simulink library "dspxfrm3"  (Simulink 6.0)
settings: Solver=ode45  SolverMode=SingleTasking  StartTime=0.0  StopTime=10.0  RelTol=1e-3
undefined symbols (not defined in the file or in its folder): D, dspblkDDClose, magnitude, Rows
libraries: dspmtrx3 x7, dspsigops x6, dspxfrm3 x6, dspsigattribs x5, dspbuff3 x2, dsparch4 x1, dspsrcs4 x1, simulink x1, dspspect3 x1
settings Model: RequirementInfo=9  CovMetricSettings=d  Creator=szlotkin  LastModifiedBy=mlongfri  ExtModeAutoUpdateStatusClock=off  ProdHWDeviceType=Specified
settings DataIOCC: SignalLoggingName=logsOut
settings OptimizationCC: BooleanDataType=off
settings DebuggingCC: CheckExecutionContextPreStartOutputMsg=on  CheckExecutionContextRuntimeOutputMsg=on  SolverPrmCheckMsg=none
settings HardwareCC: ProdHWDeviceType=Specified  TargetUnknown=on
settings ModelReferenceCC: UpdateModelReferenceTargets=IfOutOfDate
settings SFSimCC: SFSimApplyToAllLibs=on  SFSimBuildMode=Incremental

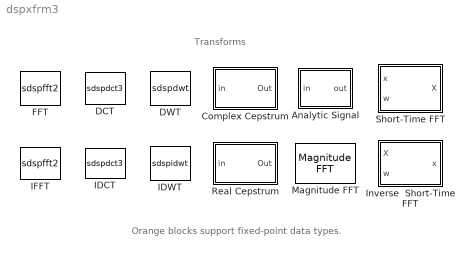
== system dspxfrm3 ==
  note: Transforms
  note: Orange blocks support fixed-point data types.
  Analytic Signal : Subsystem  PropExecContextAcrossSSBoundary=on  mask(Analytic Signal){N=100}
      mask prompts: N "Filter order (must be even):"
      mask help: Complex analytic signal of input.
      mask init:
      | x = [0,NaN,100,NaN,[58 58],NaN,[24 92],NaN,[58 24 24 58],NaN,[58 64 68 72 76 80 84 88],NaN, [42 42],NaN,[8 76],NaN,[72 68 64 60 56 52 48 42 36 32 28 24 20 16 12],NaN,[32 43 45 43 35]];
      | y = [0,NaN,100,NaN,[43 8],NaN,[16 16],NaN,[18 18 17 17],NaN,[16 24 36 24 28 28 32 16],NaN, [92 56],NaN,[64 64],NaN,[64 80 76 76 72 84 72 64 72 84 72 76 76 80 64],NaN,[51 33 41 33 35] ];
      | b=dspblkanalytic2('design',N);
      mask Help: web(dspbhelp);
      mask Display: plot(x,y)
  Complex Cepstrum : Subsystem  PropExecContextAcrossSSBoundary=on  mask(Complex Cepstrum){inheritFFT=on, N=64}
      mask prompts: inheritFFT "Inherit FFT length from input port dimensions"; N "FFT length:"
      mask help: Complex cepstrum of input signal. Input is modified to remove possible phase discontinuity at +/- pi radians.
      mask init:
      | dspblkcceps('init');
      mask Help: web(dspbhelp);
      mask CallbackString: dspblkcceps|
      mask Display: disp('Complex\n Cepstrum')
  DCT : S-Function  FunctionName=sdspdct3  Parameters=0, CompMethod  mask(DCT){CompMethod=Table lookup}
      mask prompts: CompMethod "Sine and cosine computation:"
      mask help:
      | Outputs the discrete cosine transform (DCT) of a real or complex input by computing a fast cosine transform (FCT) using a radix-2 FFT.
      |
      | Computes the DCT along the vector dimension for sample-based vector inputs, which must have a power-of-2 length. Computes the DCT along each column for all other inputs, where the columns must be a power-of-2 length.
      mask Help: web(dspbhelp);
      mask StyleString: popup(Table lookup|Trigonometric fcn)
      mask Display: disp(' DCT')
  DWT : S-Function  FunctionName=sdspdwt  Parameters=phl, phh, NumLevels, tree, Output  mask(DWT){Wname=User-defined, OrdRec_ordDec=[1 / 1], Order=2, LPF=[0.0352   -0.0854   -0.1350   0.4599   0.8069   0.3327], HPF=[-0.3327    0.8069   -0.4599   -0.1350    0.0854    0.0352], NumLevels=2, tree=Asymmetric, Output=Single port}
      mask prompts: Wname "Filter:"; OrdRec_ordDec "Filter order [synthesis / analysis]:"; Order "Wavelet order:"; LPF "Lowpass FIR filter coefficients:"; HPF "Highpass FIR filter coefficients:"; NumLevels "Number of levels:"; tree "Tree structure:"
      mask help:
      | Computes the discrete wavelet transform (DWT). Uses a filter bank with specified highpass and lowpass FIR filters to decompose the input into subbands that have smaller bandwidths and slower sample rates. The filters can be user-defined or wavelet-based (use of wavelets requires the Wavelet Toolbox).  Usually, the highpass and lowpass filters should be half-band filters designed to complement each other.
      |
      | When 'Output' is set to 'Multiple ports' the block outputs each subband from a different port as a frame-based vector or matrix (the topmost port outputs the subband with the highest frequency band). When 'Output' is set to 'Single port' the block outputs one sample-based vector or matrix of concatenated subbands.
      |
      | Inputs must be frame-based with a frame size a multiple of 2^n, where n is the value entered in the 'Number of levels.'  To create a filter bank that accepts sample-based inputs and inputs of other sizes, use Two-Channel Analysis Subband Filter blocks in the Multirate Filters library.
      |
      | This block is the same as the Dyadic Analysis Filter Bank block in the Multirate Filters library.
      mask init:
      | [x,y, str] = dspblkdwt('icon');
      | [phl, phh] = dspblkdwt('init', LPF, HPF, tree);
      mask Help: web(dspbhelp);
      mask StyleString: popup(User-defined|Haar|Daubechies|Symlets|Coiflets|Biorthogonal|Reverse Biorthogonal|Discrete Meyer),popup([1 / 1]|[1 / 3]|[1 / 5]|[2 / 2]|[2 / 4]|[2 / 6]|[2 / 8]|[3 / 1]|[3 / 3]|[3 / 5]|[3 / 7]|[3 / 9]|[4 / 4]|[5 / 5]|[6 / 8]),edit,edit,edit,edit,popup(Asymmetric|Symmetric),popup(Single port|Multiple ports)
      mask CallbackString: dspblkdwt|||||||
      mask Display:
      | disp(' DWT')
      | 
      | text(0.07,0.16,str)
  FFT : S-Function  DialogController=dspDDGCreate  DialogControllerArgs=DataTag2  FunctionName=sdspfft2  Parameters=0,CompMethod,TableOpt,BitRevOrder,0,SkipNorm,dtInfo.firstCoeffMode,dtInfo.firstCoeffWordLength,dtInfo.firstCoeffFracLength,dtInfo.prodOutputMode,dtInfo.prodOutputWordLength,dtInfo.prodOutputFracLength,dtInfo.accumMode,dtInfo.accumWordLength,dtInfo.accumFracLength,dtInfo.outputMode,dtInfo.outputWordLength,dtInfo.outputFracLength,dtInfo.roundingMode,dtInfo.overflowMode  mask(FFT){CompMethod=Table lookup, TableOpt=Speed, BitRevOrder=off, additionalParams=off, SkipNorm=on, allowOverrides=on, firstCoeffMode=Same word length as input, firstCoeffWordLength=16, firstCoeffFracLength=15, outputMode=Inherit via internal rule, outputWordLength=16, outputFracLength=15, accumMode=Inherit via internal rule, accumWordLength=32, accumFracLength=30, prodOutputMode=Inherit via internal rule, prodOutputWordLength=32, prodOutputFracLength=30, roundingMode=Floor, overflowMode=off, LockScale=off}
      mask prompts: CompMethod "Twiddle factor computation:"; TableOpt "Optimize table for:"; BitRevOrder "Output in bit-reversed order"; additionalParams "---------- Show additional parameters ----------"; SkipNorm "Skip divide-by-two on butterfly outputs for fixed-point signals"; allowOverrides "Allow overrides from DSP Fixed-Point Attributes blocks"; firstCoeffMode "Fixed-point sine table attributes:"; firstCoeffWordLength "Sine table word length:"; firstCoeffFracLength "Sine table fraction length:"; outputMode "Fixed-point output attributes:"; outputWordLength "Output word length:"; outputFracLength "Output fraction length:"; accumMode "Fixed-point accumulator attributes:"; accumWordLength "Accumulator word length:"; accumFracLength "Accumulator fraction length:"; prodOutputMode "Fixed-point product output attributes:"; prodOutputWordLength "Product output word length:"; prodOutputFracLength "Product output fraction length:"; roundingMode "Round integer calculations toward:"; overflowMode "Saturate on integer overflow"; LockScale "Lock scaling"
      mask help:
      | Outputs the complex fast Fourier transform (FFT) of a real or complex input by computing radix-2 decimation-in-time (DIT) or decimation-in-frequency (DIF), depending on block options. Uses half-length and double-signal algorithms for real inputs where possible.
      |
      | Computes the FFT along the vector dimension for sample-based vector inputs, which must have a power-of-2 length. Computes the FFT along each column for all other inputs, where the columns must be a power-of-2 length.
      mask init:
      | dtInfo = dspGetFixptDataTypeInfo(gcbh,47);
      settings: CopyFcn=dspfixptcopycallback
      mask Help: web(dspbhelp);
      mask StyleString: popup(Trigonometric fcn|Table lookup),popup(Speed|Memory),checkbox,checkbox,checkbox,checkbox,popup(Same word length as input|Specify word length|Same as input|Same as output|User-defined|Binary point scaling|Slope and bias scaling),edit,edit,popup(Inherit via internal rule|Same as input|Binary point scaling|Slope and bias scaling|User-defined),edit,edit,popup(Inherit via internal rule|Same as product output|Same as input|Binary point scaling|Slope and bias scaling|User-defined),edit,edit,popup(Inherit via internal rule|Same as input|Binary point scaling|Slope and bias scaling|User-defined),edit,edit,popup(Floor|Nearest),checkbox,checkbox
      mask Display: disp('  FFT ');
  IDCT : S-Function  FunctionName=sdspdct3  Parameters=1, CompMethod  mask(IDCT){CompMethod=Table lookup}
      mask prompts: CompMethod "Sine and cosine computation:"
      mask help:
      | Outputs the inverse discrete cosine transform (IDCT) of a real or complex input by computing an inverse fast cosine transform (IFCT) using a radix-2 IFFT.
      |
      | Computes the IDCT along the vector dimension for sample-based vector inputs, which must have a power-of-2 length. Computes the IDCT along each column for all other inputs, where the columns must be a power-of-2 length.
      mask Help: web(dspbhelp);
      mask StyleString: popup(Table lookup|Trigonometric fcn)
      mask Display: disp('IDCT')
  IDWT : S-Function  FunctionName=sdspidwt  Parameters=phl, phh, NumLevels, tree, Input  mask(IDWT){Wname=User-defined, OrdRec_ordDec=[1 / 1], Order=2, LPF=[0.3327    0.8069    0.4599   -0.1350   -0.0854    0.0352], HPF=[0.0352    0.0854   -0.1350   -0.4599    0.8069   -0.3327], NumLevels=2, tree=Asymmetric, Input=Single port}
      mask prompts: Wname "Filter:"; OrdRec_ordDec "Filter order [synthesis, analysis]:"; Order "Wavelet order:"; LPF "Lowpass FIR filter coefficients:"; HPF "Highpass FIR filter coefficients:"; NumLevels "Number of levels:"; tree "Tree Structure:"
      mask help:
      | Computes the inverse discrete wavelet transform (IDWT). Uses a filter bank with specified highpass and lowpass FIR filters to reconstruct the original signal from its subbands, which have smaller bandwidths and slower sample rates. Filters can be user-defined or wavelet-based (use of wavelets requires the Wavelet Toolbox). Usually, the highpass and lowpass filters should be half-band filters designed to complement each other.
      |
      | When 'Input' is set to 'Multiple ports', you must input each subband through a different input port as a frame-based vector or matrix (the topmost input port should receive the subband with the highest frequency band). When 'Input' is set to 'Single port', the block input must be a sample-based vector or matrix of concatenated subbands.
      |
      | To create a filter bank with less constraints on whether the inputs are frame-based or sample-based, use Two-Channel Synthesis Subband Filter blocks in the Multirate Filters library.
      |
      | This block is the same as the Dyadic Synthesis Filter Bank block in the Multirate Filters library.
      mask init:
      | [x,y,str] = dspblkidwt('icon');
      | [phl, phh] = dspblkidwt('init', LPF, HPF, tree);
      mask Help: web(dspbhelp);
      mask StyleString: popup(User-defined|Haar|Daubechies|Symlets|Coiflets|Biorthogonal|Reverse Biorthogonal|Discrete Meyer),popup([1 / 1]|[1 / 3]|[1 / 5]|[2 / 2]|[2 / 4]|[2 / 6]|[2 / 8]|[3 / 1]|[3 / 3]|[3 / 5]|[3 / 7]|[3 / 9]|[4 / 4]|[5 / 5]|[6 / 8]),edit,edit,edit,edit,popup(Asymmetric|Symmetric),popup(Single port|Multiple ports)
      mask CallbackString: dspblkidwt|||||||
      mask Display:
      | disp(' IDWT')
      | text(0.07,0.16,str)
  IFFT : S-Function  DialogController=dspDDGCreate  DialogControllerArgs=DataTag3  ClipboardFcn=dspblkDDClose;  FunctionName=sdspfft2  Parameters=1,CompMethod,TableOpt,BitRevOrder,cs_in,SkipNorm,dtInfo.firstCoeffMode,dtInfo.firstCoeffWordLength,dtInfo.firstCoeffFracLength,dtInfo.prodOutputMode,dtInfo.prodOutputWordLength,dtInfo.prodOutputFracLength,dtInfo.accumMode,dtInfo.accumWordLength,dtInfo.accumFracLength,dtInfo.outputMode,dtInfo.outputWordLength,dtInfo.outputFracLength,dtInfo.roundingMode,dtInfo.overflowMode  mask(IFFT){CompMethod=Table lookup, TableOpt=Speed, BitRevOrder=off, cs_in=off, SkipNorm=off, mode=Complex, additionalParams=off, allowOverrides=on, firstCoeffMode=Same word length as input, firstCoeffWordLength=16, firstCoeffFracLength=15, outputMode=Inherit via internal rule, outputWordLength=16, outputFracLength=15, accumMode=Inherit via internal rule, accumWordLength=32, accumFracLength=30, prodOutputMode=Inherit via internal rule, prodOutputWordLength=32, prodOutputFracLength=30, roundingMode=Floor, overflowMode=off, LockScale=off}
      mask prompts: CompMethod "Twiddle factor computation:"; TableOpt "Optimize table for:"; BitRevOrder "Input is in bit-reversed order"; cs_in "Input is conjugate symmetric"; SkipNorm "Skip scaling"; mode "Output:"; additionalParams "---------- Show additional parameters ----------"; allowOverrides "Allow overrides from DSP FPA Fixed-Point Attributes blocks"; firstCoeffMode "Fixed-point sine table attributes:"; firstCoeffWordLength "Sine table word length:"; firstCoeffFracLength "Sine table fraction length:"; outputMode "Fixed-point output attributes:"; outputWordLength "Output word length:"; outputFracLength "Output fraction length:"; accumMode "Fixed-point accumulator attributes:"; accumWordLength "Accumulator word length:"; accumFracLength "Accumulator fraction length:"; prodOutputMode "Fixed-point product output attributes:"; prodOutputWordLength "Product output word length:"; prodOutputFracLength "Product output fraction length:"; roundingMode "Round integer calculations toward:"; overflowMode "Saturate on integer overflow"; LockScale "Lock scaling"
      mask help:
      | Outputs the inverse fast Fourier transform (IFFT) of a real or complex input by computing radix-2 decimation-in-time (DIT) or decimation-in-frequency (DIF), depending on block options. Outputs are real if you select 'Input is conjugate symmetric' option; otherwise, outputs are complex.
      |
      | Computes the IFFT along the vector dimension for sample-based vector inputs, which must have a power-of-2 length. Computes the IFFT along each column for all other inputs, where the columns must be a power-of-2 length.
      mask init:
      | dtInfo = dspGetFixptDataTypeInfo(gcbh,47);
      settings: CopyFcn=dspfixptcopycallback
      mask Help: web(dspbhelp);
      mask StyleString: popup(Trigonometric fcn|Table lookup),popup(Speed|Memory),checkbox,checkbox,checkbox,popup(Real|Complex),checkbox,checkbox,popup(Same word length as input|Specify word length|Same as input|Same as output|User-defined|Binary point scaling|Slope and bias scaling),edit,edit,popup(Inherit via internal rule|Same as input|Binary point scaling|Slope and bias scaling|User-defined),edit,edit,popup(Inherit via internal rule|Same as product output|Same as input|Binary point scaling|Slope and bias scaling|User-defined),edit,edit,popup(Inherit via internal rule|Same as input|Binary point scaling|Slope and bias scaling|User-defined),edit,edit,popup(Floor|Nearest),checkbox,checkbox
      mask Display: disp('  IFFT')
  Inverse  Short-Time FFT : Subsystem  PropExecContextAcrossSSBoundary=on  mask(Inverse Short-Time FFT){OvLap=512-16, OutFrameSize=512, InConjSymm=on, DoAssert=off, W=512, Tol=1e-4}
      mask prompts: OvLap "Overlap between consecutive STFFT frames (in samples):"; OutFrameSize "Samples per output frame:"; InConjSymm "Input is conjugate symmetric"; DoAssert "Assert if analysis window does not support perfect signal reconstruction"; W "Analysis window length:"; Tol "Reconstruction error tolerance:"
      mask help:
      | Reconstructs a signal from its Short-Time FFT (STFFT) by using the OLA method. The block takes as an input the analysis window w[n] used in the generation of the STFFT to normalize the output signal.
      |
      | Optionally, the block asserts if the analysis window does not satisfy
      | constraints that permit perfect reconstruction of the signal.
      mask init:
      | L = dspblkistfft('init',DoAssert,OvLap,W,InConjSymm);
      mask Help: web(dspbhelp)
      mask CallbackString: |||dspblkistfft('dynamic');||
      mask Display:
      | port_label('input',1,'X[nL,k]')
      | port_label('output',1,'x[n]')
      | port_label('input',2,'w[n]')
  Magnitude FFT : dspspect3/Magnitude FFT  mag_or_magsq=Magnitude squared  fftLenInherit=off  fftsize=256
  Real Cepstrum : Subsystem  PropExecContextAcrossSSBoundary=on  mask(Real Cepstrum){inheritFFT=on, N=64}
      mask prompts: inheritFFT "Inherit FFT length from input port dimensions"; N "FFT length:"
      mask help: Real cepstrum of input signal.
      mask init:
      | dspblkrceps('init');
      mask Help: web(dspbhelp);
      mask CallbackString: dspblkrceps|
      mask Display: disp('Real\nCepstrum')
  Short-Time FFT : Subsystem  PropExecContextAcrossSSBoundary=on  mask(Short-Time FFT){W=512, OvLap=512-16, M=1024}
      mask prompts: W "Analysis window length:"; OvLap "Overlap between consecutive windows (in samples):"; M "FFT length:"
      mask help:
      | Output the Short-Time FFT of the input signal x[n].
      | Uses an externally specified analysis window w[n].
      mask init:
      | L = W-OvLap;
      settings: CopyFcn=dspfixptcopycallback
      mask Help: web(dspbhelp)
      mask Display:
      | port_label('input',1,'x[n]')
      | port_label('input',2,'w[n]')
      | port_label('output',1,'X[nL,k]')

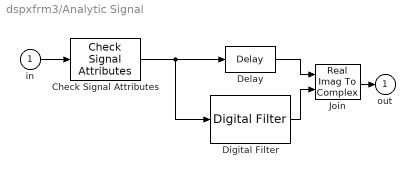
== system dspxfrm3/Analytic Signal ==
  in : Inport  LatchInput=off
  Check Signal Attributes : dspsigattribs/Check Signal Attributes  SigAttribCheckMethod=Does not match attributes exactly  Complexity=Ignore  Frame=Ignore  DimsCheckMethod=Ignore  Dimensions=1-D  DatatypeCheckMethod=Is...  DatatypeGeneral=Floating-point  DtypeFloatSpecific=Any floating-point  DtypeFixedSpecific=Any fixed-point  DtypeIntSpecific=Any integer  SampleMode=Ignore
  Delay : dspsigops/Delay  dly_unit=Samples  delay=N/2  ic_detail=off  dif_ic_for_ch=off  dif_ic_for_dly=off  ic=0  reset_popup=None
  Digital Filter : dsparch4/Digital Filter  TypePopup=FIR (all zeros)  IIRFiltStruct=Direct form II transposed  AllPoleFiltStruct=Direct form  FIRFiltStruct=Direct form transposed  CoeffSource=Specify via dialog  NumCoeffs=b  DenCoeffs=[1 0.1]  BiQuadCoeffs=[1 0.3 0.4 1 0.1 0.2]  LatticeCoeffs=[0.2 0.4]  denIgnore=on  FiltPerSampPopup=One filter per frame  IC=0  ICnum=0  ICden=0  roundingMode=Floor  overflowMode=off
  Join : RealImagToComplex
  out : Outport  InitialOutput=0
  wires:
  Digital Filter/1 -> Join/2
  Delay/1 -> Join/1
  Join/1 -> out/1
  in/1 -> Check Signal Attributes/1
  Check Signal Attributes/1 -> Delay/1, Digital Filter/1

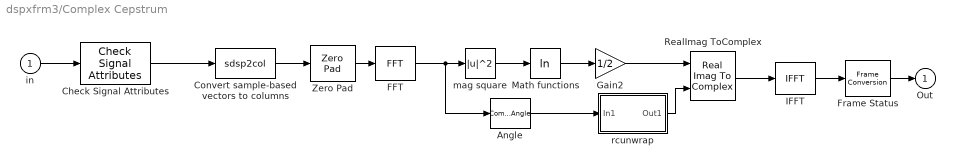
== system dspxfrm3/Complex Cepstrum ==
  in : Inport  LatchInput=off
  Angle : ComplexToMagnitudeAngle  Output=Angle
  Check Signal Attributes : dspsigattribs/Check Signal Attributes  SigAttribCheckMethod=Does not match attributes exactly  Complexity=Real  Frame=Ignore  DimsCheckMethod=Ignore  Dimensions=1-D  DatatypeCheckMethod=Is...  DatatypeGeneral=Floating-point  DtypeFloatSpecific=Any floating-point  DtypeFixedSpecific=Any fixed-point  DtypeIntSpecific=Any integer  SampleMode=Discrete
  Convert sample-based vectors to columns : S-Function  FunctionName=sdsp2col
  FFT : dspxfrm3/FFT  DialogController=dspDDGCreate  DialogControllerArgs=DataTag0  CompMethod=Table lookup  TableOpt=Speed  BitRevOrder=off  SkipNorm=on  roundingMode=Floor  overflowMode=off
  Frame Status : FrameConversion  OutFrame=Sample based
  Gain2 : Gain  Gain=1/2  SaturateOnIntegerOverflow=on
  IFFT : dspxfrm3/IFFT  DialogController=dspDDGCreate  DialogControllerArgs=DataTag1  CompMethod=Table lookup  TableOpt=Speed  BitRevOrder=off  cs_in=on  SkipNorm=off  mode=Real  roundingMode=Floor  overflowMode=off
  Math functions : Math  Operator=log  SaturateOnIntegerOverflow=on
  RealImag ToComplex : RealImagToComplex
  Zero Pad : dspsigops/Zero Pad  padSigAt=End  zpadAlong=None  padNumOutRowsSpecMethod=User-specified  numOutRows=N  padNumOutColsSpecMethod=User-specified  numOutCols=1  trunc_flag=None
  mag square : Math  Operator=magnitude^2  SaturateOnIntegerOverflow=on
  rcunwrap : Subsystem  PropExecContextAcrossSSBoundary=on
  Out : Outport  InitialOutput=0
  wires:
  Gain2/1 -> RealImag ToComplex/1
  rcunwrap/1(Out1) -> RealImag ToComplex/2
  mag square/1 -> Math functions/1
  Math functions/1 -> Gain2/1
  in/1 -> Check Signal Attributes/1
  FFT/1 -> mag square/1, Angle/1
  Angle/1 -> rcunwrap/1(In1)
  IFFT/1 -> Frame Status/1
  Convert sample-based vectors to columns/1 -> Zero Pad/1
  Zero Pad/1 -> FFT/1
  Frame Status/1 -> Out/1
  RealImag ToComplex/1 -> IFFT/1
  Check Signal Attributes/1 -> Convert sample-based vectors to columns/1

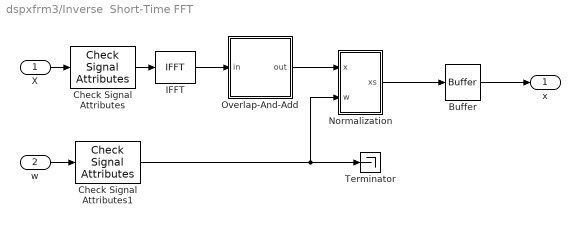
== system dspxfrm3/Inverse  Short-Time FFT ==
  X : Inport  LatchInput=off
  w : Inport  Port=2  LatchInput=off
  Buffer : dspbuff3/Buffer  N=OutFrameSize  V=0  ic=0
  Check Signal Attributes : dspsigattribs/Check Signal Attributes  SigAttribCheckMethod=Does not match attributes exactly  Complexity=Ignore  Frame=Ignore  DimsCheckMethod=Ignore  Dimensions=1-D  DatatypeCheckMethod=Is...  DatatypeGeneral=Floating-point  DtypeFloatSpecific=Any floating-point  DtypeFixedSpecific=Any fixed-point  DtypeIntSpecific=Any integer  SampleMode=Ignore
  Check Signal Attributes1 : dspsigattribs/Check Signal Attributes  SigAttribCheckMethod=Does not match attributes exactly  Complexity=Ignore  Frame=Ignore  DimsCheckMethod=Ignore  Dimensions=1-D  DatatypeCheckMethod=Is...  DatatypeGeneral=Floating-point  DtypeFloatSpecific=Any floating-point  DtypeFixedSpecific=Any fixed-point  DtypeIntSpecific=Any integer  SampleMode=Ignore
  IFFT : dspxfrm3/IFFT  DialogController=dspDDGCreate  DialogControllerArgs=DataTag4  CompMethod=Table lookup  TableOpt=Speed  BitRevOrder=off  cs_in=on  SkipNorm=off  mode=Real  roundingMode=Floor  overflowMode=off
  Normalization : Subsystem  PropExecContextAcrossSSBoundary=on
  Overlap-And-Add : Subsystem  PropExecContextAcrossSSBoundary=on  mask(Overlap-And-Add){L=L}
      mask prompts: L "Number of new points in each frame"
      mask help: Performs overlap-and-add on the input signal. Disjoint frames of the input signal are overlapped with each other for a specified number of points and summed.
      mask Display: disp('Overlap\nAnd\nAdd')
  Terminator : Terminator
  x : Outport
  wires:
  Normalization/1(xs) -> Buffer/1
  IFFT/1 -> Overlap-And-Add/1(in)
  Overlap-And-Add/1(out) -> Normalization/1(x)
  X/1 -> Check Signal Attributes/1
  w/1 -> Check Signal Attributes1/1
  Buffer/1 -> x/1
  Check Signal Attributes/1 -> IFFT/1
  Check Signal Attributes1/1 -> Normalization/2(w), Terminator/1

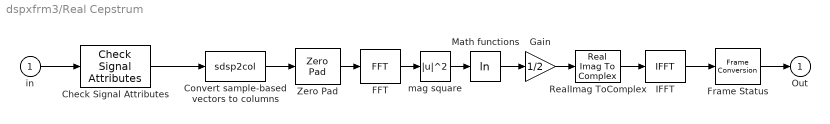
== system dspxfrm3/Real Cepstrum ==
  in : Inport  LatchInput=off
  Check Signal Attributes : dspsigattribs/Check Signal Attributes  SigAttribCheckMethod=Does not match attributes exactly  Complexity=Real  Frame=Ignore  DimsCheckMethod=Ignore  Dimensions=1-D  DatatypeCheckMethod=Is...  DatatypeGeneral=Floating-point  DtypeFloatSpecific=Any floating-point  DtypeFixedSpecific=Any fixed-point  DtypeIntSpecific=Any integer  SampleMode=Discrete
  Convert sample-based vectors to columns : S-Function  FunctionName=sdsp2col
  FFT : dspxfrm3/FFT  DialogController=dspDDGCreate  DialogControllerArgs=DataTag5  CompMethod=Table lookup  TableOpt=Speed  BitRevOrder=off  SkipNorm=on  roundingMode=Floor  overflowMode=off
  Frame Status : FrameConversion  OutFrame=Sample based
  Gain : Gain  Gain=1/2  SaturateOnIntegerOverflow=on
  IFFT : dspxfrm3/IFFT  DialogController=dspDDGCreate  DialogControllerArgs=DataTag6  CompMethod=Table lookup  TableOpt=Speed  BitRevOrder=off  cs_in=on  SkipNorm=off  mode=Real  roundingMode=Floor  overflowMode=off
  Math functions : Math  Operator=log  SaturateOnIntegerOverflow=on
  RealImag ToComplex : RealImagToComplex  Input=Real
  Zero Pad : dspsigops/Zero Pad  padSigAt=End  zpadAlong=None  padNumOutRowsSpecMethod=User-specified  numOutRows=N  padNumOutColsSpecMethod=User-specified  numOutCols=1  trunc_flag=None
  mag square : Math  Operator=magnitude^2  SaturateOnIntegerOverflow=on
  Out : Outport  InitialOutput=0
  wires:
  Zero Pad/1 -> FFT/1
  in/1 -> Check Signal Attributes/1
  FFT/1 -> mag square/1
  mag square/1 -> Math functions/1
  Math functions/1 -> Gain/1
  Gain/1 -> RealImag ToComplex/1
  IFFT/1 -> Frame Status/1
  Convert sample-based vectors to columns/1 -> Zero Pad/1
  Frame Status/1 -> Out/1
  RealImag ToComplex/1 -> IFFT/1
  Check Signal Attributes/1 -> Convert sample-based vectors to columns/1

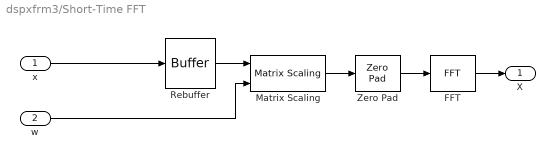
== system dspxfrm3/Short-Time FFT ==
  x : Inport  LatchInput=off
  w : Inport  Port=2  LatchInput=off
  FFT : dspxfrm3/FFT  DialogController=dspDDGCreate  DialogControllerArgs=DataTag7  CompMethod=Table lookup  TableOpt=Speed  BitRevOrder=off  SkipNorm=on  roundingMode=Floor  overflowMode=off
  Matrix Scaling : dspmtrx3/Matrix Scaling  DialogController=dspDDGCreate  DialogControllerArgs=DataTag8  mode=Scale rows (D*A)  D_Source=Input port  D_VectFromMask=[0.5 0.25]  roundingMode=Floor  overflowMode=off
  Rebuffer : dspbuff3/Buffer  N=W  V=W-L  ic=0
  Zero Pad : dspsigops/Zero Pad  padSigAt=End  zpadAlong=Columns  padNumOutRowsSpecMethod=User-specified  numOutRows=M  padNumOutColsSpecMethod=User-specified  numOutCols=1  trunc_flag=None
  X : Outport
  wires:
  FFT/1 -> X/1
  w/1 -> Matrix Scaling/2
  x/1 -> Rebuffer/1
  Matrix Scaling/1 -> Zero Pad/1
  Zero Pad/1 -> FFT/1
  Rebuffer/1 -> Matrix Scaling/1

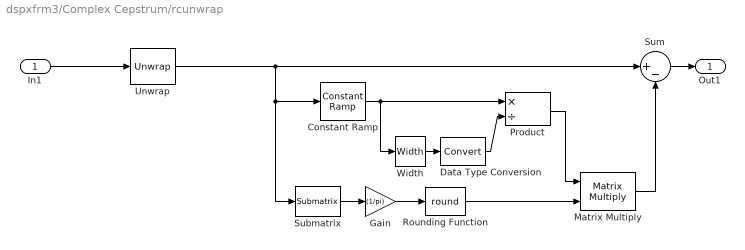
== system dspxfrm3/Complex Cepstrum/rcunwrap ==
  In1 : Inport  LatchInput=off
  Constant Ramp : dspsrcs4/Constant Ramp  L=Rows  Slope=2*pi  Offset=0
  Data Type Conversion : DataTypeConversion  SaturateOnIntegerOverflow=on  RndMeth=Zero
  Gain : Gain  Gain=(1/pi)  SaturateOnIntegerOverflow=on
  Matrix Multiply : dspmtrx3/Matrix Multiply  numInputPorts=2  OptimizationLevel=None
  Product : Product  Inputs=*/  SaturateOnIntegerOverflow=on  InputSameDT=on
  Rounding Function : Rounding  Operator=round
  Submatrix : dspmtrx3/Submatrix  RowSpan=One row  RowStartMode=Middle  RowStartIndex=1  RowEndMode=Last  RowEndIndex=1  ColSpan=All columns  ColStartMode=First  ColStartIndex=1  ColEndMode=Last  ColEndIndex=1
  Sum : Sum  Inputs=|+-  SaturateOnIntegerOverflow=on  InputSameDT=on
  Unwrap : dspsigops/Unwrap  running=on  tol=pi
  Width : Width  DataType=int32
  Out1 : Outport
  wires:
  In1/1 -> Unwrap/1
  Sum/1 -> Out1/1
  Rounding Function/1 -> Matrix Multiply/2
  Gain/1 -> Rounding Function/1
  Submatrix/1 -> Gain/1
  Unwrap/1 -> Sum/1, Constant Ramp/1, Submatrix/1
  Matrix Multiply/1 -> Sum/2
  Constant Ramp/1 -> Product/1, Width/1
  Product/1 -> Matrix Multiply/1
  Data Type Conversion/1 -> Product/2
  Width/1 -> Data Type Conversion/1

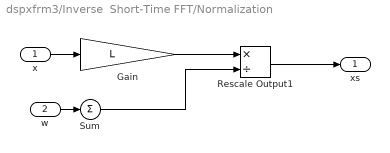
== system dspxfrm3/Inverse  Short-Time FFT/Normalization ==
  x : Inport  LatchInput=off
  w : Inport  Port=2  LatchInput=off
  Gain : Gain  Gain=L  SaturateOnIntegerOverflow=on
  Rescale Output1 : Product  Inputs=*/  InputSameDT=on
  Sum : Sum  Inputs=+  SaturateOnIntegerOverflow=on
  xs : Outport
  wires:
  Gain/1 -> Rescale Output1/1
  Sum/1 -> Rescale Output1/2
  w/1 -> Sum/1
  Rescale Output1/1 -> xs/1
  x/1 -> Gain/1

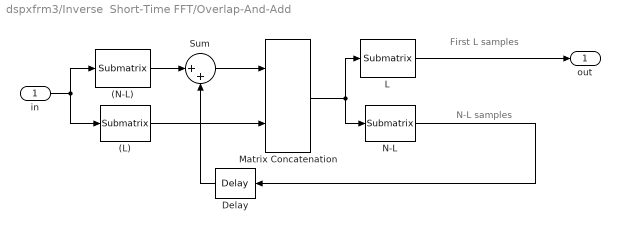
== system dspxfrm3/Inverse  Short-Time FFT/Overlap-And-Add ==
  note: N-L samples
  note: First L samples
  in : Inport  LatchInput=off
  (L) : dspmtrx3/Submatrix  RowSpan=Range of rows  RowStartMode=Offset from last  RowStartIndex=L-1  RowEndMode=Last  RowEndIndex=1  ColSpan=All columns  ColStartMode=First  ColStartIndex=1  ColEndMode=Last  ColEndIndex=1
  (N-L) : dspmtrx3/Submatrix  RowSpan=Range of rows  RowStartMode=First  RowStartIndex=1  RowEndMode=Offset from last  RowEndIndex=L  ColSpan=All columns  ColStartMode=First  ColStartIndex=1  ColEndMode=Last  ColEndIndex=1
  Delay : dspsigops/Delay  Orientation=left  dly_unit=Frames  delay=1  ic_detail=off  dif_ic_for_ch=off  dif_ic_for_dly=off  ic=0  reset_popup=None
  L : dspmtrx3/Submatrix  RowSpan=Range of rows  RowStartMode=First  RowStartIndex=1  RowEndMode=Index  RowEndIndex=L  ColSpan=All columns  ColStartMode=First  ColStartIndex=1  ColEndMode=Last  ColEndIndex=1
  Matrix Concatenation : simulink/Math Operations/Matrix Concatenation  numInports=2  catMethod=Vertical
  N-L : dspmtrx3/Submatrix  RowSpan=Range of rows  RowStartMode=Index  RowStartIndex=L+1  RowEndMode=Last  RowEndIndex=1  ColSpan=All columns  ColStartMode=First  ColStartIndex=1  ColEndMode=Last  ColEndIndex=1
  Sum : Sum  Inputs=|++  SaturateOnIntegerOverflow=on  InputSameDT=on
  out : Outport
  wires:
  in/1 -> (N-L)/1, (L)/1
  Matrix Concatenation/1 -> N-L/1, L/1
  N-L/1 -> Delay/1
  (L)/1 -> Matrix Concatenation/2
  Delay/1 -> Sum/2
  (N-L)/1 -> Sum/1
  Sum/1 -> Matrix Concatenation/1
  L/1 -> out/1
